simulink subsystem "VectorExpand"  (R2022b)
settings: Solver=VariableStepAuto  StartTime=0.0  StopTime=10.0  RelTol=1e-3
Description:
  | Copyright (c) 2023, Alexei Evsenin, evsenin@gmail.com
settings Model: Creator=evsenin  LastModifiedBy=evsenin
settings ModelReferenceCC: EnableRefExpFcnMdlSchedulingChecks=on

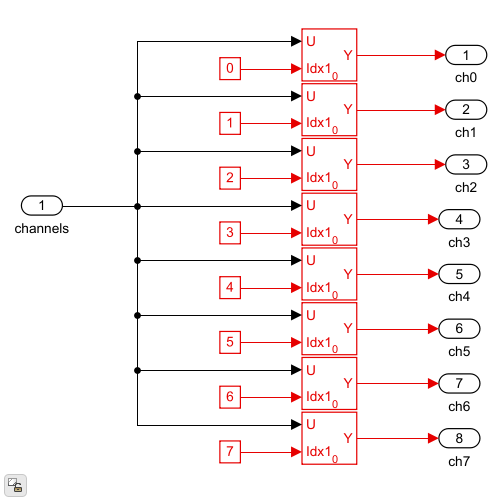
[thumbnail: Simulink's stored preview of the top-level diagram]
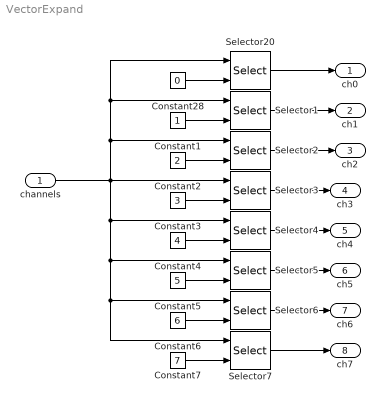
== system VectorExpand ==
  channels : Inport
  Constant1 : Constant  OutDataTypeStr=uint8  SampleTime=-1
  Constant2 : Constant  Value=2  OutDataTypeStr=uint8  SampleTime=-1
  Constant28 : Constant  Value=0  OutDataTypeStr=uint8  SampleTime=-1
  Constant3 : Constant  Value=3  OutDataTypeStr=uint8  SampleTime=-1
  Constant4 : Constant  Value=4  OutDataTypeStr=uint8  SampleTime=-1
  Constant5 : Constant  Value=5  OutDataTypeStr=uint8  SampleTime=-1
  Constant6 : Constant  Value=6  OutDataTypeStr=uint8  SampleTime=-1
  Constant7 : Constant  Value=7  OutDataTypeStr=uint8  SampleTime=-1
  Selector{1..7,20} (8 alike) : Selector  IndexMode=Zero-based  IndexOptions=Index vector (port)  Indices=[1 3]  OutputSizes=1
  ch0 : Outport
  ch1 : Outport  Port=2
  ch2 : Outport  Port=3
  ch3 : Outport  Port=4
  ch4 : Outport  Port=5
  ch5 : Outport  Port=6
  ch6 : Outport  Port=7
  ch7 : Outport  Port=8
  wires:
  Constant28/1 -> Selector20/2
  Selector20/1 -> ch0/1
  Constant1/1 -> Selector1/2
  Selector1/1 -> ch1/1
  Constant2/1 -> Selector2/2
  Selector2/1 -> ch2/1
  Selector3/1 -> ch3/1
  Constant3/1 -> Selector3/2
  Selector4/1 -> ch4/1
  Constant4/1 -> Selector4/2
  Selector5/1 -> ch5/1
  Constant5/1 -> Selector5/2
  Selector6/1 -> ch6/1
  Constant6/1 -> Selector6/2
  Selector7/1 -> ch7/1
  channels/1 -> Selector20/1, Selector1/1, Selector2/1, Selector3/1, Selector4/1, Selector5/1, Selector6/1, Selector7/1
  Constant7/1 -> Selector7/2
